simulink model "sim1"  (R2024b)
settings: Solver=ode1  StartTime=0.0  StopTime=30  FixedStep=1/1440  RelTol=1e-3
settings Model: Creator=yugpn  LastModifiedBy=yugpn

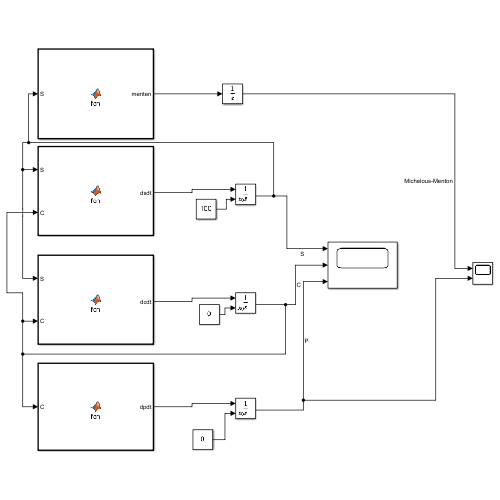
[thumbnail: Simulink's stored preview of the top-level diagram]
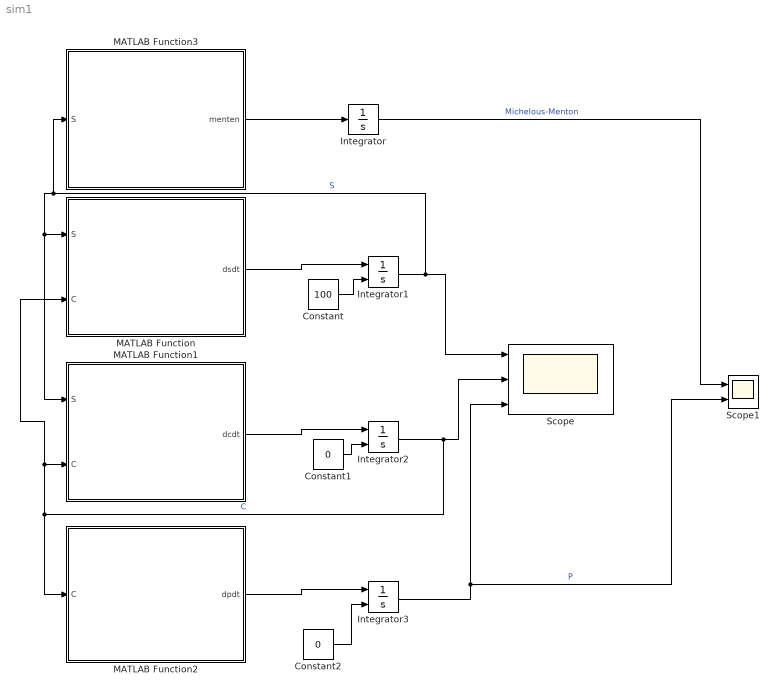
== system sim1 ==
  Constant : Constant  Value=100
  Constant1 : Constant  Value=0
  Constant2 : Constant  Value=0
  Integrator : Integrator
  Integrator1 : Integrator  InitialConditionSource=external
  Integrator2 : Integrator  InitialConditionSource=external
  Integrator3 : Integrator  InitialConditionSource=external
  MATLAB Function : MATLAB Function  TreatAsAtomicUnit=on
  MATLAB Function1 : MATLAB Function  TreatAsAtomicUnit=on
  MATLAB Function2 : MATLAB Function  TreatAsAtomicUnit=on
  MATLAB Function3 : MATLAB Function  TreatAsAtomicUnit=on
  Scope : Scope  NumInputPorts=3
  Scope1 : Scope  NumInputPorts=2
  wires:
  MATLAB Function3/1(menten) -> Integrator/1
  MATLAB Function/1(dsdt) -> Integrator1/1
  MATLAB Function1/1(dcdt) -> Integrator2/1
  MATLAB Function2/1(dpdt) -> Integrator3/1
  Constant/1 -> Integrator1/2
  Constant1/1 -> Integrator2/2
  Constant2/1 -> Integrator3/2
  Integrator2/1 -> MATLAB Function/2(C), MATLAB Function1/2(C), MATLAB Function2/1(C), Scope/2  "C"
  Integrator3/1 -> Scope/3, Scope1/2  "P"
  Integrator/1 -> Scope1/1  "Michelous-Menton"
  Integrator1/1 -> MATLAB Function3/1(S), MATLAB Function1/1(S), MATLAB Function/1(S), Scope/1  "S"

== matlab function sim1/MATLAB Function ==
  data: S input; dsdt output; C input
function dsdt = fcn(S, C)

dsdt =(-0.1724*S)*(10-C)+0.01724*C ;

== matlab function sim1/MATLAB Function2 ==
  data: C input; dpdt output
function dpdt = fcn(C)

dpdt = C*0.5;

== matlab function sim1/MATLAB Function3 ==
  data: S input; menten output
function menten = fcn(S)

menten = (5*S)/(0.1724+S);

== matlab function sim1/MATLAB Function1 ==
  data: S input; dcdt output; C input
function dcdt = fcn(S, C)

dcdt = (0.1724*S)*(10-C)-(0.01724+0.5)*C;
